simulink model "surus_cevrimi"  (R2020b)
settings: Solver=VariableStepAuto  StartTime=0  StopTime=drive_time  RelTol=1e-3
values from neighbouring files (symbols this model uses):
  A = 2.27    [electric_vehicle_edit.m]
  bat_capacity = 36*36*(10^5)    (= 129600000)    [electric_vehicle_edit.m]
  bat_eff = 0.92    [electric_vehicle_edit.m]
  cd = 0.28    [electric_vehicle_edit.m]
  f = 0.01    [electric_vehicle_edit.m]    (also in spring_eq_code.m = 2)
  g = 9.81    [electric_vehicle_edit.m]
  m = 5    [diff_equiations_code.m]    (also in electric_vehicle_edit.m = 1500; spring_eq_code.m = 2)
  me = 1.02*m    (= 1530)    [electric_vehicle_edit.m]
  p_aksesuar = 4000    [electric_vehicle_edit.m]
  r_int = 0.1    [electric_vehicle_edit.m]
  ro_air = 1.2    [electric_vehicle_edit.m]
  rw = 0.32    [electric_vehicle_edit.m]
  transmission = 7.524    [electric_vehicle_edit.m]
  v_ocv = 350    [electric_vehicle_edit.m]
undefined symbols (not defined in the file or in its folder): eff_map, sigbuilder_block
libraries: simulink x4, autolibshared x1, pid_lib x1
settings Model: Creator=amnessa  LastModifiedBy=amnessa

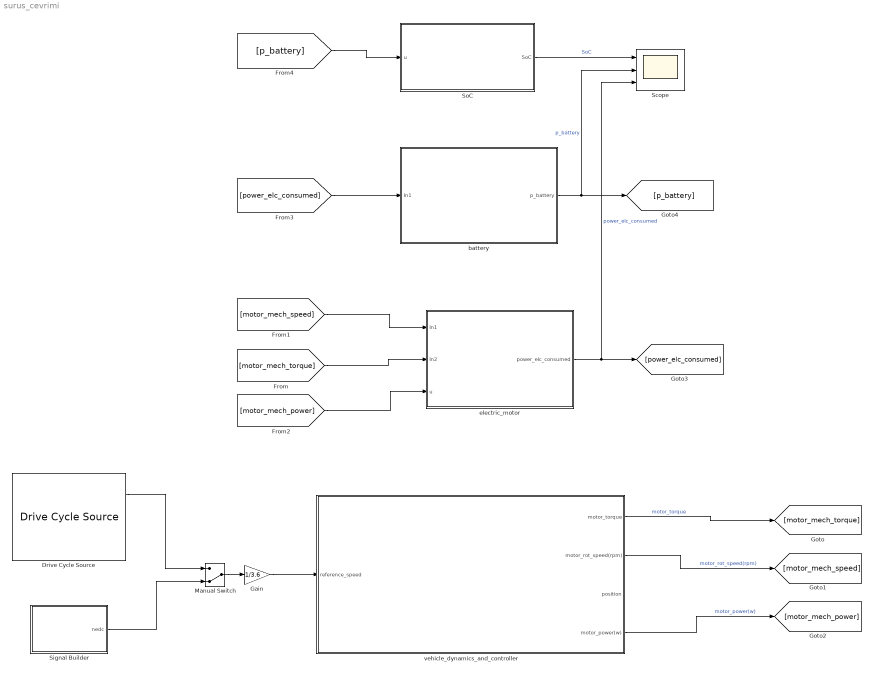
== system surus_cevrimi ==
  Drive Cycle Source : autolibshared/Drive Cycle Source  cycleVar=.mat, .xls, .xlsx or .txt file  fileVar=C:\Users\amnessa\Desktop\Matlab_simulink_projects\simulink_kurs_tüm_dosyalar\bölüm7_elektrikli_tasıt\drive_cycle_and_effmap\wltp.xlsx  tfinal="1800  seconds"  cycleRepeat=off  outAccPort=on  outGearPort=off  gearList=No gear data  t_wot1=5  xdot_woto=0  xdot_wot1=30  t_wot2=20  xdot_wot2=0  t_wotend=30  srcUnit=km/h  outUnit=km/h  srcAccUnit=km/h/s  outAccUnit=m/s^2  dt=0  aMode=1  faultOption=off  velBnd=2  velBndUnit=mph  inUnit=m/s  timeBnd=1  failOption=off  stopSim=off  maxFaultCnt=10  maxFaultTime=2  maxTotFaultTime=15  traceOption=off  dtTrace=1  traceWindow=10  lastDCname=Custom Data Set  lastOutUnit=mph  lastDT=0  lastTB=1  lastSB=2  forceCalcBound=off
      settings: SourceProductBaseCode=PW,MT,UV,VE,VP
  Gain : Gain  Gain=1/3.6
  Manual Switch : ManualSwitch  CurrentSetting=0
  Scope : Scope  NumInputPorts=3
  Signal Builder : Subsystem  Tag=STV Subsys  LoadFcn=sigbuilder_block('load');  StartFcn=sigbuilder_block('start');  StopFcn=sigbuilder_block('stop');  ClipboardFcn=sigbuilder_block('clipboard');  mask(Sigbuilder block){tuvar=[0:10]}
      mask help: Simulink:masks:SigbuilderBlock_MD
      mask init:
      | if ~strcmp(get_param(bdroot(gcbh),'SimulationStatus'),'stopped') tuvar = sigbuilder_block('maskInit'); end
      settings: CopyFcn=sigbuilder_block('copy');  DeleteFcn=sigbuilder_block('delete');  ModelCloseFcn=sigbuilder_block('modelClose');  PreSaveFcn=sigbuilder_block('preSave');  PauseFcn=sigbuilder_block('pause');  ContinueFcn=sigbuilder_block('continue');  NameChangeFcn=sigbuilder_block('namechange');  OpenFcn=sigbuilder_block('open',[0 30 1440 722.25 ]);  CloseFcn=sigbuilder_block('close');
      mask Display: plot(0, 0, 100, 100,[2, 2, 32, 32, 2], [68, 8, 8, 68, 68],[32, 2], [38, 38], [32, 19, 2],[53, 60, 44], [32, 17, 17, 2],[16, 16, 31, 31]);txt = getActiveGroup(gcbh);text(2, 100, txt,'verticalAlignment', 'top');
  SoC : Subsystem
      mask Display: image('C:\Users\amnessa\Desktop\Matlab_simulink_projects\simulink_kurs_tüm_dosyalar\bölüm7_elektrikli_tasıt\görsel\Measuring_Your_State_Of_Charge.jpg'); % Use "Edit Image" on toolstrip to change.
  battery : Subsystem
      mask Display: image('C:\Users\amnessa\Desktop\Matlab_simulink_projects\simulink_kurs_tüm_dosyalar\bölüm7_elektrikli_tasıt\görsel\Screenshot (411).png'); % Use "Edit Image" on toolstrip to change.
  electric_motor : Subsystem
      mask Display: image('C:\Users\amnessa\Desktop\Matlab_simulink_projects\simulink_kurs_tüm_dosyalar\bölüm7_elektrikli_tasıt\görsel\DC-motor-parts.png'); % Use "Edit Image" on toolstrip to change.
  vehicle_dynamics_and_controller : Subsystem
      mask Display: image('C:\Users\amnessa\Desktop\Matlab_simulink_projects\simulink_kurs_tüm_dosyalar\bölüm7_elektrikli_tasıt\görsel\Nissan_Leaf_2018-17.jpg'); % Use "Edit Image" on toolstrip to change.
  wires:
  Drive Cycle Source/1 -> Manual Switch/1
  Signal Builder/1(nedc) -> Manual Switch/2
  Manual Switch/1 -> Gain/1
  Gain/1 -> vehicle_dynamics_and_controller/1(reference_speed)
  vehicle_dynamics_and_controller/1(motor_torque) -> [motor_mech_torque]  "motor_torque"
  vehicle_dynamics_and_controller/2(motor_rot_speed(rpm)) -> [motor_mech_speed]  "motor_rot_speed(rpm)"
  vehicle_dynamics_and_controller/4(motor_power(w)) -> [motor_mech_power]  "motor_power(w)"
  [motor_mech_speed] -> electric_motor/1(In1)
  [motor_mech_torque] -> electric_motor/2(In2)
  [motor_mech_power] -> electric_motor/3(u)
  electric_motor/1(power_elc_consumed) -> Scope/3, [power_elc_consumed]  "power_elc_consumed"
  [power_elc_consumed] -> battery/1(In1)
  battery/1(p_battery) -> Scope/2, [p_battery]  "p_battery"
  [p_battery] -> SoC/1(u)
  SoC/1(SoC) -> Scope/1  "SoC"

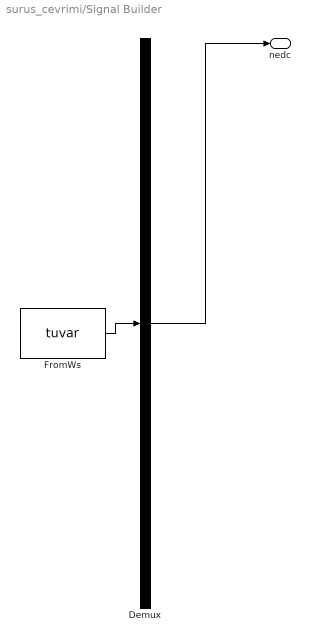
== system surus_cevrimi/Signal Builder ==
  Demux : Demux  Tag=STV Demux  Outputs=1
      settings: DisplayOption=none
  FromWs : FromWorkspace  Tag=STV FromWs  VariableName=tuvar
      SigBuilderData=|
      | common.afterFinalStr = 'Extrapolate'
      | common.sampleTime = 0
      | dataSet.timeRange = [0 1180]
      | dataSet.name = 'Group 1'
      | sbobj.Groups.Name = 'Group 1'
      | sbobj.Groups.Signals.Name = 'nedc'
      | sbobj.Groups.Signals.XData = [0 2 3 4 5 6 7 8 9 10 11 12 ... (1180 elements, 1x1180)]
      | sbobj.Groups.Signals.YData = [0 0 0 0 0 0 0 0 0 0 0 3.8 ... (1180 elements, 1x1180)]
      | sbobj.Groups.TimeRange = [0 1180]
  nedc : Outport  Tag=STV Outport
  wires:
  Demux/1 -> nedc/1
  FromWs/1 -> Demux/1

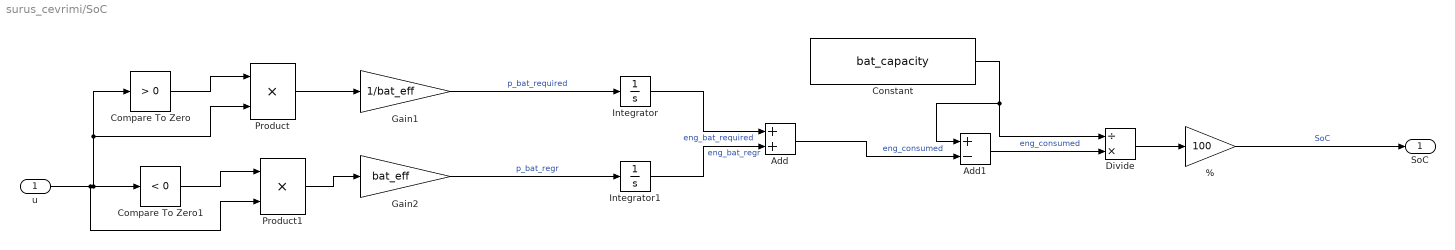
== system surus_cevrimi/SoC ==
  u : Inport
  % : Gain  Gain=100
  Add : Sum
  Add1 : Sum  Inputs=+-
  Compare To Zero : simulink/Logic and Bit Operations/Compare To Zero  relop=>  OutDataTypeStr=boolean
  Compare To Zero1 : simulink/Logic and Bit Operations/Compare To Zero  relop=<  OutDataTypeStr=boolean
  Constant : Constant  Value=bat_capacity
  Divide : Product  Inputs=/*
  Gain1 : Gain  Gain=1/bat_eff
  Gain2 : Gain  Gain=bat_eff
  Integrator : Integrator
  Integrator1 : Integrator
  Product : Product
  Product1 : Product
  SoC : Outport
  wires:
  Constant/1 -> Divide/1, Add1/1
  Compare To Zero/1 -> Product/1
  Divide/1 -> %/1
  u/1 -> Compare To Zero1/1, Product/2, Compare To Zero/1, Product1/2
  Product1/1 -> Gain2/1
  Gain1/1 -> Integrator/1  "p_bat_required"
  Gain2/1 -> Integrator1/1  "p_bat_regr"
  Integrator/1 -> Add/1  "eng_bat_required"
  Compare To Zero1/1 -> Product1/1
  Add1/1 -> Divide/2  "eng_consumed"
  Product/1 -> Gain1/1
  Integrator1/1 -> Add/2  "eng_bat_regr"
  Add/1 -> Add1/2  "eng_consumed"
  %/1 -> SoC/1  "SoC"

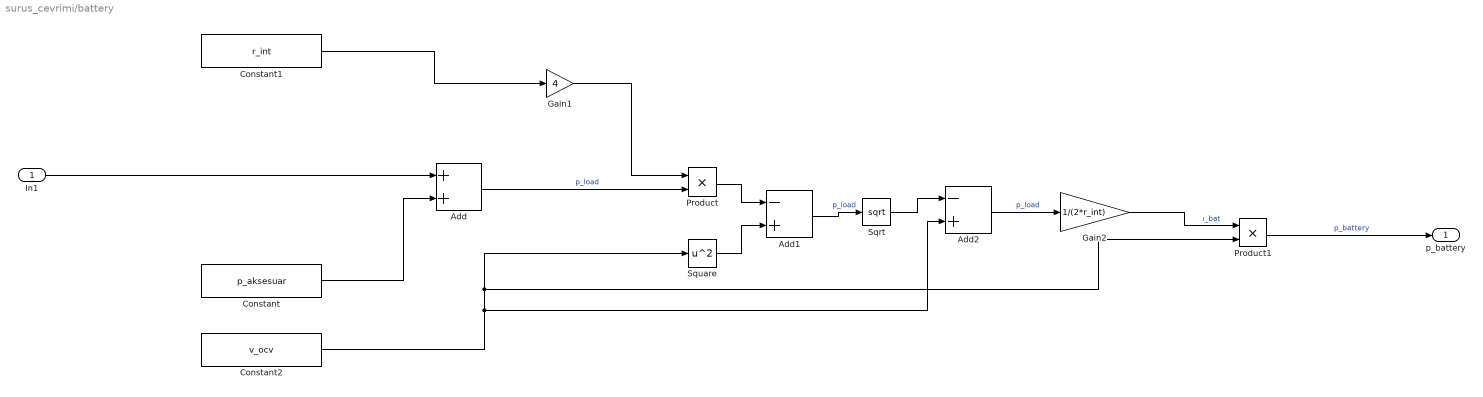
== system surus_cevrimi/battery ==
  In1 : Inport
  Add : Sum
  Add1 : Sum  Inputs=-+
  Add2 : Sum  Inputs=-+
  Constant : Constant  Value=p_aksesuar
  Constant1 : Constant  Value=r_int
  Constant2 : Constant  Value=v_ocv
  Gain1 : Gain  Gain=4
  Gain2 : Gain  Gain=1/(2*r_int)
  Product : Product
  Product1 : Product
  Sqrt : Sqrt  SaturateOnIntegerOverflow=on
  Square : Math  Operator=square  SaturateOnIntegerOverflow=on
  p_battery : Outport
  wires:
  Constant2/1 -> Product1/2, Square/1, Add2/2
  Square/1 -> Add1/2
  Add/1 -> Product/2  "p_load"
  Product1/1 -> p_battery/1  "p_battery"
  Gain1/1 -> Product/1
  Product/1 -> Add1/1
  Sqrt/1 -> Add2/1
  Add2/1 -> Gain2/1  "p_load"
  Constant1/1 -> Gain1/1
  Add1/1 -> Sqrt/1  "p_load"
  Gain2/1 -> Product1/1  "ı_bat"
  Constant/1 -> Add/2
  In1/1 -> Add/1

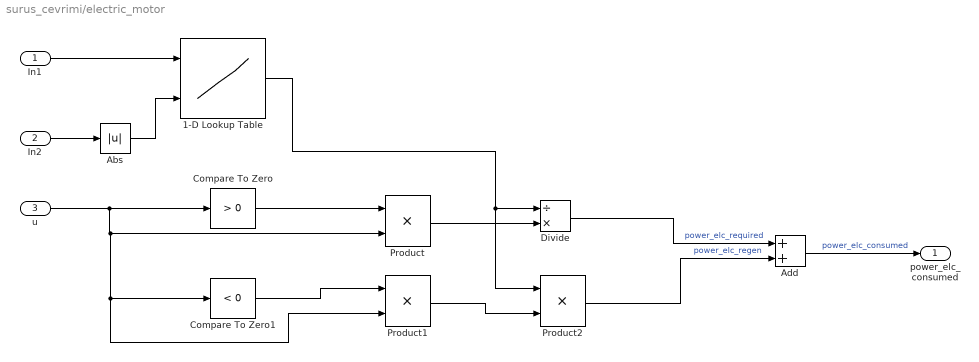
== system surus_cevrimi/electric_motor ==
  In1 : Inport
  In2 : Inport  Port=2
  u : Inport  Port=3
  1-D Lookup Table : Lookup_n-D  BreakpointsForDimension1=eff_map.speed  BreakpointsForDimension2=eff_map.torque  Table=eff_map.efficiency  InternalRulePriority=Speed  RndMeth=Simplest  InputSameDT=on
      settings: InputPortMap=u0,u1
  Abs : Abs
  Add : Sum
  Compare To Zero : simulink/Logic and Bit Operations/Compare To Zero  relop=>  OutDataTypeStr=boolean
  Compare To Zero1 : simulink/Logic and Bit Operations/Compare To Zero  relop=<  OutDataTypeStr=boolean
  Divide : Product  Inputs=/*
  Product : Product
  Product1 : Product
  Product2 : Product
  power_elc_consumed : Outport
  wires:
  Compare To Zero/1 -> Product/1
  1-D Lookup Table/1 -> Product2/1, Divide/1
  Product/1 -> Divide/2
  Divide/1 -> Add/1  "power_elc_required"
  u/1 -> Product1/2, Compare To Zero1/1, Product/2, Compare To Zero/1
  Product2/1 -> Add/2  "power_elc_regen"
  Compare To Zero1/1 -> Product1/1
  Product1/1 -> Product2/2
  Abs/1 -> 1-D Lookup Table/2
  In2/1 -> Abs/1
  In1/1 -> 1-D Lookup Table/1
  Add/1 -> power_elc_consumed/1  "power_elc_consumed"

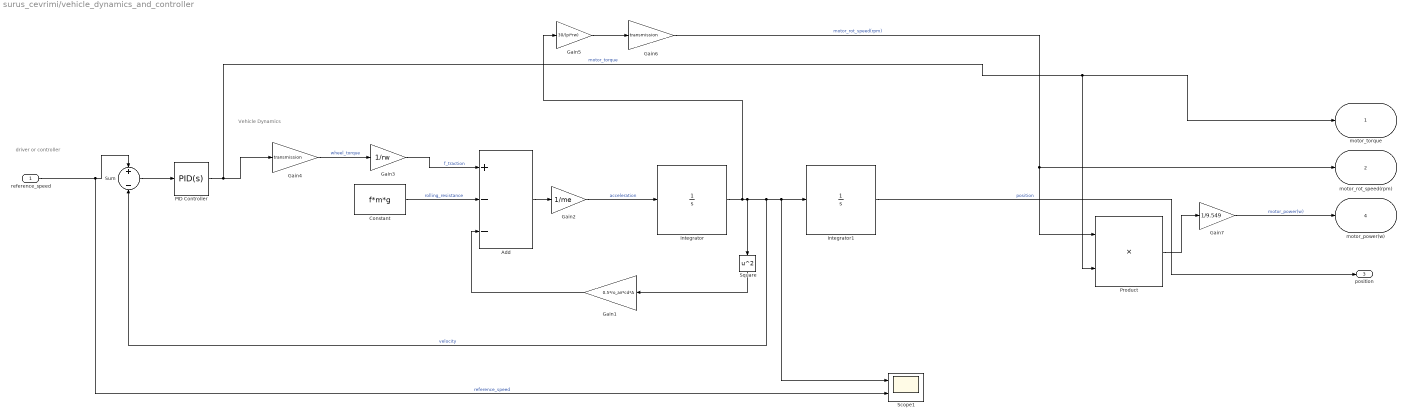
== system surus_cevrimi/vehicle_dynamics_and_controller ==
  note: driver or controller
  note: Vehicle Dynamics
  reference_speed : Inport
  Add : Sum  Inputs=+--
  Constant : Constant  Value=f*m*g
  Gain1 : Gain  Gain=0.5*ro_air*cd*A
  Gain2 : Gain  Gain=1/me
  Gain3 : Gain  Gain=1/rw
  Gain4 : Gain  Gain=transmission
  Gain5 : Gain  Gain=30/(pi*rw)
  Gain6 : Gain  Gain=transmission
  Gain7 : Gain  Gain=1/9.549
  Integrator : Integrator
  Integrator1 : Integrator
  PID Controller : pid_lib/PID Controller  Controller=PID  Form=Parallel  TimeDomain=Continuous-time  UseExternalTs=off  SampleTime=-1  IntegratorMethod=Forward Euler  FilterMethod=Forward Euler  ControllerParametersSource=internal  P=620.656823334484  I=1096.26740706283  D=11.7869770659031  UseFilter=on  N=36.46824066771  TunerSelectOption=Transfer Function Based (PID Tuner App)  InitialConditionSource=internal  InitialConditionForIntegrator=0  InitialConditionForFilter=0  DifferentiatorICPrevScaledInput=0  ExternalReset=none  TrackingMode=off  Kt=1  LimitOutput=off  SatLimitsSource=internal  UpperSaturationLimit=inf  LowerSaturationLimit=-inf  LinearizeAsGain=on  AntiWindupMode=none  Kb=1  POutMin=[]  POutMax=[]  IOutMin=[]  IOutMax=[]  DOutMin=[]  DOutMax=[]  NOutMin=[]  NOutMax=[]  SumOutMin=[]  SumOutMax=[]  SaturationOutMin=[]  SaturationOutMax=[]  PParamMin=[]  PParamMax=[]  IParamMin=[]  IParamMax=[]  DParamMin=[]  DParamMax=[]  NParamMin=[]  NParamMax=[]  KbParamMin=[]  KbParamMax=[]  KtParamMin=[]  KtParamMax=[]  KbOutMin=[]  KbOutMax=[]  KtOutMin=[]  KtOutMax=[]  IntegratorOutMin=[]  IntegratorOutMax=[]  FilterOutMin=[]  FilterOutMax=[]  SumI1OutMin=[]  SumI1OutMax=[]  SumI2OutMin=[]  SumI2OutMax=[]  SumI3OutMin=[]  SumI3OutMax=[]  SumI4OutMin=[]  SumI4OutMax=[]  SumDOutMin=[]  SumDOutMax=[]  DifferentiatorOutMin=[]  DifferentiatorOutMax=[]  FilterDiffOutCoefMin=[]  FilterDiffOutCoefMax=[]  ReciprocalOutMin=[]  ReciprocalOutMax=[]  SumDenOutMin=[]  SumDenOutMax=[]  SumNumOutMin=[]  SumNumOutMax=[]  DivideOutMin=[]  DivideOutMax=[]  UdiffTsProdOutMin=[]  UdiffTsProdOutMax=[]  NTsProdOutMin=[]  NTsProdOutMax=[]  UintegralTsProdOutMin=[]  UintegralTsProdOutMax=[]  UngainTsProdOutMin=[]  UngainTsProdOutMax=[]  IntegratorContinuousStateAttributes=''  IntegratorStateMustResolveToSignalObject=off  IntegratorRTWStateStorageClass=Auto  FilterContinuousStateAttributes=''  FilterStateMustResolveToSignalObject=off  FilterRTWStateStorageClass=Auto  ParallelPVariant=InternalParameters  IdealPVariant=Disabled  IVariant=InternalParameters  DVariant=InternalParameters  IntegratorVariant=Continuous  SatVariant=Disabled  AWVariant=Passthrough  PCopyVariant=Disabled  TRVariant=Disabled  FdbkBlocksVariant=Forward  IdealPFdbkVariant=Disabled  SatFdbkVariant=Disabled  DerivativeFilterVariant=ContFilter  NVariant=InternalParameters  NCopyVariant=Disabled  FilterICVariant=InternalICsFilter  IntegratorICVariant=InternalICs  ExternalResetVariant=Disabled  TRSumVariant=Passthrough  SumFdbkVariant=Disabled  SumVariant=Sum_PID  TsampFilterVariant=InternalTs  TsampNgainVariant=Passthrough  TsampIntegralVariant=Passthrough  ExternalSaturationOutDataTypeStr=Inherit: Same as second input
  Product : Product
  Scope1 : Scope  NumInputPorts=2
  Square : Math  Operator=square  SaturateOnIntegerOverflow=on
  Sum : Sum  Inputs=+-
  motor_torque : Outport
  motor_rot_speed(rpm) : Outport  Port=2
  position : Outport  Port=3
  motor_power(w) : Outport  Port=4
  wires:
  Integrator/1 -> Gain5/1, Scope1/1, Integrator1/1, Sum/2, Square/1  "velocity"
  Product/1 -> Gain7/1
  Sum/1 -> PID Controller/1
  Constant/1 -> Add/2  "rolling_resistance"
  Gain4/1 -> Gain3/1  "wheel_torque"
  Gain1/1 -> Add/3
  PID Controller/1 -> motor_torque/1, Product/2, Gain4/1  "motor_torque"
  Gain6/1 -> motor_rot_speed(rpm)/1, Product/1  "motor_rot_speed(rpm)"
  Integrator1/1 -> position/1  "position"
  reference_speed/1 -> Scope1/2, Sum/1  "reference_speed"
  Gain3/1 -> Add/1  "f_traction"
  Gain7/1 -> motor_power(w)/1  "motor_power(w)"
  Gain2/1 -> Integrator/1  "acceleration"
  Add/1 -> Gain2/1
  Square/1 -> Gain1/1
  Gain5/1 -> Gain6/1
